simulink model "pipeline_observer"  (R2023a)
settings: Solver=ode45  StartTime=0.0  StopTime=200  MaxStep=0.1  RelTol=1e-3
settings Model: Creator=Theodora  LastModifiedBy=Theodora

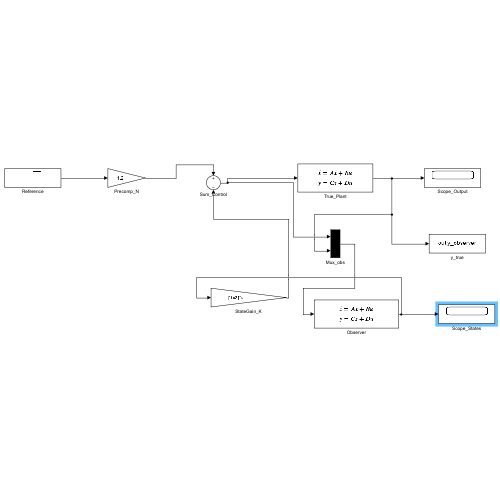
[thumbnail: Simulink's stored preview of the top-level diagram]
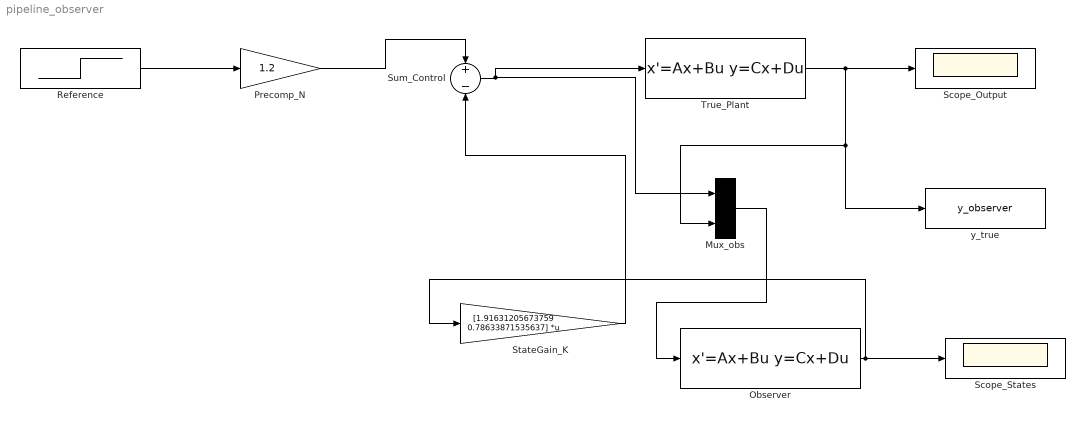
== system pipeline_observer ==
  Mux_obs : Mux  Inputs=2
  Observer : StateSpace  A=[-0.5 -9.99999999999999;1 -7]  B=[0.5 9.99999999999999;0 6.85815602836879]  C=[1 0;0 1]  D=[0 0;0 0]  InitialCondition=[0.1; 0.1]
  Precomp_N : Gain  Gain=1.2
  Reference : Step  Time=0  SampleTime=0
  Scope_Output : Scope
  Scope_States : Scope
  StateGain_K : Gain  Gain=[1.91631205673759 0.78633871535637]  Multiplication=Matrix(K*u)
  Sum_Control : Sum  Inputs=+-
  True_Plant : StateSpace  A=[-0.5 0;1 -0.141843971631206]  B=[0.5;0]  C=[0 1]  D=0  InitialCondition=[0; 0]
  y_true : ToWorkspace  VariableName=y_observer  SampleTime=-1
  wires:
  Reference/1 -> Precomp_N/1
  Precomp_N/1 -> Sum_Control/1
  Sum_Control/1 -> True_Plant/1, Mux_obs/1
  True_Plant/1 -> y_true/1, Mux_obs/2, Scope_Output/1
  Mux_obs/1 -> Observer/1
  Observer/1 -> StateGain_K/1, Scope_States/1
  StateGain_K/1 -> Sum_Control/2
